simulink model "Arrays1"  (Simulink 9.0)
settings: Solver=FixedStepDiscrete  StartTime=0.0  StopTime=19800  FixedStep=200  RelTol=1e-3  EnableMultiTasking=on
model workspace (MAT data in the model file):
  already_pp = 1
  input_dataset = Simulink.SimulationData.Dataset
  input_dataset.any.Name = ''
  input_dataset.any.Version = 3
  input_dataset.any.Storage = Simulink.SimulationData.Storage.RamDatasetStorage
  input_dataset.any.Storage.any.Version = 2
  input_dataset.any.Storage.any.Elements{1} = Simulink.SimulationData.Signal
  input_dataset.any.Storage.any.Elements{1}.Version = 1
  input_dataset.any.Storage.any.Elements{1}.Values = timeseries
  input_dataset.any.Storage.any.Elements{1}.Values.Name = 'unnamed'
  input_dataset.any.Storage.any.Elements{1}.Values.DataInfo = tsdata.datametadata
  input_dataset.any.Storage.any.Elements{1}.Values.DataInfo.Interpolation = tsdata.interpolation
  input_dataset.any.Storage.any.Elements{1}.Values.DataInfo.Interpolation.Fhandle : function handle (value not decoded)
  input_dataset.any.Storage.any.Elements{1}.Values.DataInfo.Interpolation.Name = 'linear'
  input_dataset.any.Storage.any.Elements{1}.Values.TimeInfo = tsdata.timemetadata
  input_dataset.any.Storage.any.Elements{1}.Values.TimeInfo.Length = 100
  input_dataset.any.Storage.any.Elements{1}.Values.TimeInfo.DuplicateTimes = 0
  input_dataset.any.Storage.any.Elements{1}.Values.TimeInfo.Time_ = [0; 200; 400; 600; 800; 1000; 1200; 1400; 1600; 1800; 2000; 2200; 2400; 2600; 2800; 3000; 3200; 3400; 3600; 3800; 4000; 4200; 4400; 4600; 4800; 5000; 5200; 5400; 5600; 5800; 6000; 6200; 6400; 6600; 6800; 7000; 7200; 7400; 7600; 7800; 8000; 8200; 8400; 8600; 8800; 9000; 9200; 9400; 9600; 9800; 10000; 10200; 10400; 10600; 10800; 11000; 11200; 11400; 11600; 11800; 12000; 12200; 12400; 12600; 12800; 13000; 13200; 13400; 13600; 13800; 14000; 14200; 14400; 14600; 14800; 15000; 15200; 15400; 15600; 15800; 16000; 16200; 16400; 16600; 16800; 17000; 17200; 17400; 17600; 17800; 18000; 18200; 18400; 18600; 18800; 19000; 19200; 19400; 19600; 19800]
  input_dataset.any.Storage.any.Elements{1}.Values.TimeInfo.Initialized = 1
  input_dataset.any.Storage.any.Elements{1}.Values.QualityInfo = tsdata.qualmetadata
  input_dataset.any.Storage.any.Elements{1}.Values.Data_ = [188.834211836; 243.475162245; -223.807910224; 248.025513683; 79.4155477352; -241.475757; -132.90106868; 28.128911523; 274.504101261; 278.93312112; -205.432150993; 282.355669056; 274.300168946; -8.7746107663; 180.168281333; -214.868196824; -46.9432304242; 249.441315113; 175.324397736; 275.695455836; 93.444419494; -278.572992855; 209.477583521; 260.395948655; 107.241092915; 154.644078347; 145.879480875; -64.6637882795; 93.2867341065; -197.287987313; 123.627652812; -280.900292174; -133.846209023; -272.297165621; -241.720931258; 194.074696996; 116.897173785; -109.740311963; 270.133229303; -279.332351698; -36.7533842062; -71.0649257442; 159.310072889; 177.119940682; -187.876437267; -6.14136252706; -32.6482795735; 87.7878060668; 125.618898515; 152.812009189; -134.384953801; 107.821606112; 93.0588023843; -202.432958883; -228.601391065; -0.981568810714; 275.84637511; -95.7685640003; 51.1606505879; -165.712836305; 150.760235583; -146.942930724; 3.57423099909; 119.446033594; 234.541951521; 275.574855123; 28.3293179783; -216.825334303; -210.423596665; -145.495047526; 204.43035359; -147.430692617; 188.570895641; -153.885018765; 257.558173912; -90.0097404091; -182.042849741; -149.349685214; 69.626805688; -16.0266906584; -89.0042957622; 198.497176738; 51.1584546916; 29.8341649747; 250.316198298; -128.496588708; 154.320137466; 152.237456567; -71.7324918148; 40.6929844351; -254.487426262; -267.6299288; 18.4785318054; 167.500338061; 260.406410538; -222.056274916; 41.2941965233; -18.3656153651; -292.858758299; -97.7264133607]
  input_dataset.any.Storage.any.Elements{1}.Name = 'E'
settings Model: SuppressorTable=22 serialization::archive 11 0 6 0 0 0 0 0  Creator=scaife  LastModifiedBy=hbourbou  ExtModeAutoUpdateStatusClock=off
settings DataIOCC: ExternalInput=input_dataset  LimitDataPoints=on  LoadExternalInput=on  SaveFormat=Dataset  SignalLoggingSaveFormat=ModelDataLogs  SaveState=on  SignalLoggingName=sigsOut
settings DebuggingCC: AlgebraicLoopMsg=error  ArtificialAlgebraicLoopMsg=error  SaveWithParameterizedLinksMsg=none  SignalResolutionControl=TryResolveAllWithWarning  MultiTaskDSMMsg=warning  MultiTaskCondExecSysMsg=none  StrictBusMsg=None
settings HardwareCC: TargetUnknown=on
settings SFSimCC: SimParseCustomCode=off
settings GRTTargetCC: GeneratePreprocessorConditionals=Disable all  CombineOutputUpdateFcns=off  GRTInterface=on  ExtMode=on

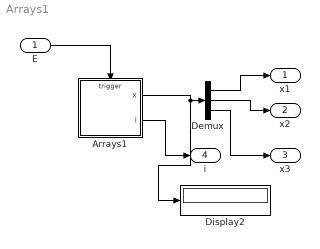
== system Arrays1 ==
  E : Inport
  Arrays1 : Stateflow chart  TreatAsAtomicUnit=on
  Demux : Demux  Outputs=3
  Display2 : Display
  x1 : Outport
  x2 : Outport  Port=2
  x3 : Outport  Port=3
  i : Outport  Port=4
  wires:
  E/1 -> Arrays1/Trigger
  Arrays1/1(x) -> Display2/1, Demux/1
  Demux/1 -> x1/1
  Demux/2 -> x2/1
  Demux/3 -> x3/1
  Arrays1/2(i) -> i/1

== stateflow chart Arrays1 ==
  state A/
    en:
    i = 1;
    x = x([3, 1, 2]) + 1;
  state B/
    en:
    i = 2;
    x([i, 1]) = x([2, 3]) + 1;
  state C/
    en:
    i = 3;
    x(3) = x(3) + 1;
  (default) -> A
  A -> B : E
  C -> A : E
  B -> C : E
  data: x output int32 size=3 [0..100] =int32([1 ;2 ;3]); i output int32 =int32(0)
  events: E input RISING_EDGE_EVENT
